simulink model "FuzzyPICon"  (Simulink 9.3)
settings: Solver=VariableStepAuto  StartTime=0.0  StopTime=10.0  RelTol=1e-3
libraries: fuzblock x1
settings Model: Creator=Kostas  LastModifiedBy=Kostas
settings DataIOCC: SaveFormat=Dataset  SignalLoggingSaveFormat=Dataset  ReturnWorkspaceOutputs=on
settings OptimizationCC: LifeSpan=auto
settings DebuggingCC: UnderspecifiedInitializationDetection=Simplified  MergeDetectMultiDrivingBlocksExec=error  FcnCallInpInsideContextMsg=error  SFUnexpectedBacktrackingDiag=error  SFNoUnconditionalDefaultTransitionDiag=error  SFExecutionAtInitializationDiag=warning  ArithmeticOperatorsInVariantConditions=error
settings HardwareCC: ProdBitPerPointer=64  ProdBitPerSizeT=64  ProdBitPerPtrDiffT=64  ProdLargestAtomicFloat=Float  ProdIntDivRoundTo=Zero  ProdEndianess=LittleEndian  ProdWordSize=64  ProdHWDeviceType=Intel->x86-64 (Windows64)
settings ModelReferenceCC: PropagateSignalLabelsOutOfModel=on
settings SFSimCC: SimUseLocalCustomCode=on
settings RTWCC: RTWUseLocalCustomCode=on
settings CodeAppCC: StateflowObjectComments=off
settings GRTTargetCC: TargetLangStandard=C99 (ISO)  CombineOutputUpdateFcns=on  GRTInterface=off
settings ConfigComp: CovMetricSettings=dwe  CovHtmlReporting=off  CovSaveCumulativeToWorkspaceVar=off  CovSaveSingleToWorkspaceVar=off  CovExternalEMLEnable=on

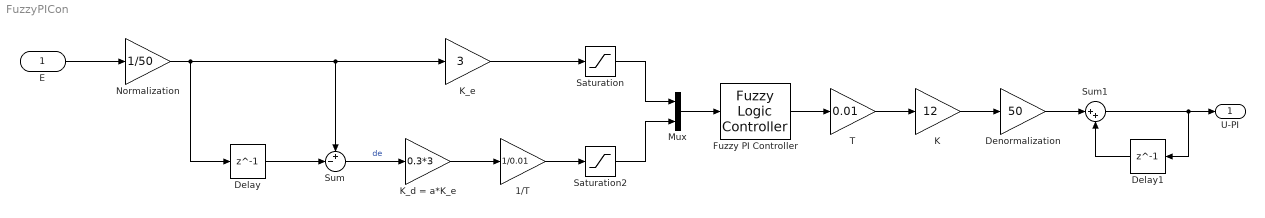
== system FuzzyPICon ==
  E : Inport
  1/T : Gain  Gain=1/0.01
  Delay : Delay  DelayLength=1  InitialCondition=0
  Delay1 : Delay  DelayLength=1  InitialCondition=0
  Denormalization : Gain  Gain=50
  Fuzzy PI Controller : fuzblock/Fuzzy Logic  Controller  FIS=fuzzyPIController.fis  OutputSampleNumber=101  DataType=double  FuzzifiedInputs=off  RuleFiringStrengths=off  RuleOutputs=off  AggregatedOutputs=off  SimulateUsing=Interpreted execution  OutOfRangeInputValueMessage=warning  NoRuleFiredMessage=warning  EmptyOutputFuzzySetMessage=warning
  K : Gain  Gain=12
  K_d = a*K_e : Gain  Gain=0.3*3
  K_e : Gain  Gain=3
  Mux : Mux  Inputs=2
  Normalization : Gain  Gain=1/50
  Saturation : Saturate
  Saturation2 : Saturate
  Sum : Sum  Inputs=+-|
  Sum1 : Sum  Inputs=|++
  T : Gain  Gain=0.01
  U-PI : Outport
  wires:
  E/1 -> Normalization/1
  Delay/1 -> Sum/2
  Normalization/1 -> Delay/1, Sum/1, K_e/1
  Sum/1 -> K_d = a*K_e/1  "de"
  K_d = a*K_e/1 -> 1/T/1
  1/T/1 -> Saturation2/1
  K_e/1 -> Saturation/1
  Saturation/1 -> Mux/1
  Saturation2/1 -> Mux/2
  Mux/1 -> Fuzzy PI Controller/1
  Fuzzy PI Controller/1 -> T/1
  T/1 -> K/1
  K/1 -> Denormalization/1
  Denormalization/1 -> Sum1/1
  Delay1/1 -> Sum1/2
  Sum1/1 -> Delay1/1, U-PI/1
